simulink model "EKF_CodeOptimiert"  (Simulink 8.0)
settings: Solver=ode1  StartTime=0.0  StopTime=Inf  FixedStep=0.001  RelTol=1e-3
undefined symbols (not defined in the file or in its folder): d_p1, d_p2, g, l_1, l_2, m_1, m_2, m_3, P, Q, R, T, x0
settings Model: Creator=Bosselmann  LastModifiedBy=Bosselmann  BufferReuse=off
settings OptimizationCC: BlockReduction=off  OptimizeBlockIOStorage=off  BufferReuse=off  ExpressionFolding=off  LocalBlockOutputs=off
settings HardwareCC: ProdIntDivRoundTo=Zero  ProdEndianess=BigEndian  ProdHWDeviceType=Generic->Custom  TargetIntDivRoundTo=Zero  TargetEndianess=BigEndian  TargetHWDeviceType=Generic->Custom
settings RTWCC: SystemTargetFile=rti1401.tlc  MakeCommand=make_rti  TemplateMakefile=rti1401.tmf  Description=dSPACE DS1401 Hardware Platform  ProcessScript=rti1401_make_rtw_hook
settings STFCustomTargetCC: CodeReplacementLibrary=ANSI_C  ParMdlRefBuildCompliant=on  GeneratePreprocessorConditionals=Disable all  MatFileLogging=on  SystemTargetFile=rti1401.tlc
settings GRTTargetCC: CompOptLevelCompliant=off  ConcurrentExecutionCompliant=off  CombineOutputUpdateFcns=off  GRTInterface=on
settings CustomProperty: DataType=RTWOptions_EnumType_C__Program Files (x86)_dSPACE RCPHIL 74_MATLAB_RTI_RTI1401_TLC_rti1401_1InitialSimState  Value=RUN
settings EnumStrPairs: String=RUN

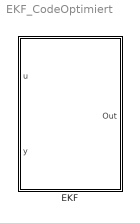
== system EKF_CodeOptimiert ==
  EKF : Subsystem

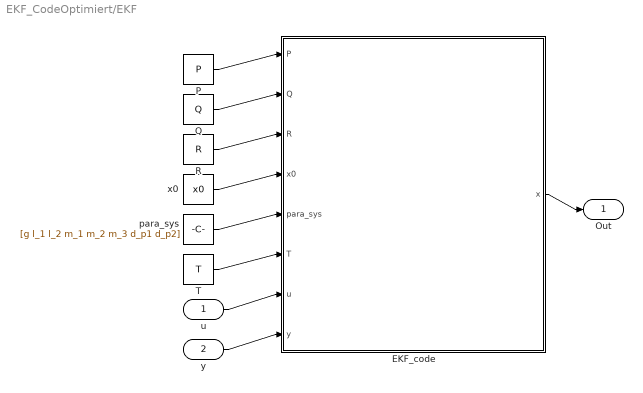
== system EKF_CodeOptimiert/EKF ==
  u : Inport
  y : Inport  Port=2
  EKF_code : MATLAB Function  TreatAsAtomicUnit=on
  P : Constant  Value=P
  Q : Constant  Value=Q
  R : Constant  Value=R
  T : Constant  Value=T
  para_sys : Constant  Value=[g l_1 l_2 m_1 m_2 m_3 d_p1 d_p2]
  x0 : Constant  Value=x0
  Out : Outport
  wires:
  P/1 -> EKF_code/1(P)
  Q/1 -> EKF_code/2(Q)
  R/1 -> EKF_code/3(R)
  x0/1 -> EKF_code/4(x0)
  para_sys/1 -> EKF_code/5(para_sys)
  T/1 -> EKF_code/6(T)
  u/1 -> EKF_code/7(u)
  y/1 -> EKF_code/8(y)
  EKF_code/1(x) -> Out/1

== matlab function EKF/EKF_code ==
  data: P input double; Q input double; R input double; x0 input double; para_sys input double; T input double; u input double; y input double; x output double
function x  = extended_kalman_filter(P, Q, R, x0, para_sys, T, u, y)
% Extended Kalman Filter (EKF) fuer nichtlineare Systeme
% Das Extended Kalman Filter praediziert den Zustand eines nichtlinearen
% Systems durch Linearisierung im Arbeistpunkt.
% R ist die Kovarianzmatrix fuer das Messrauschen.
% Q ist die Kovarianzmatrix fuer das Prozessrauschen.
% Das Verhaeltnis von Q und R gibt die Dynamik des Filters vor.

persistent x_p P_p
% Parameter

g = para_sys(1);
l_1 = para_sys(2);
l_2 = para_sys(3);
m_1 = para_sys(4);
m_2 = para_sys(5);
m_3 = para_sys(6);
d_p1 = para_sys(7);
d_p2 = para_sys(8);

if isempty(x_p)
   x_p = x0;
   P_p = P;
   x = x_p;
else
%% Discrete Kalman filter time update equations

 x_1 = x_p(1);
 x_2 = x_p(2);
 x_3 = x_p(3);
 x_4 = x_p(4);

  t3 = x_1-x_3;
  t2 = cos(t3);
  t4 = cos(x_1);
  t5 = sin(x_1);
  t6 = sin(t3);
  t7 = l_1^2;
  t8 = x_2^2;
  t9 = m_2^2;
  t10 = cos(x_3);
  t11 = sin(x_3);
  t12 = l_2^2;
  t13 = x_4^2;
  t14 = x_1*2.0;
  t15 = t14-x_3*2.0;
  t16 = t14-x_3;
  t17 = cos(t16);
  t18 = sin(t16);
  t1 = zeros(4,1);
  t1(1,1) = x_1+T*x_2;
  t1(2,1) = x_2+(T*1.0/l_1^2*(-t2*(d_p2*l_1*x_2*1.8e1-d_p2*l_1*x_4*1.8e1+g*l_1*l_2*m_2*t11*9.0+l_1*l_2*m_2*t10*u*9.0+l_2*m_2*t6*t7*t8*9.0)-d_p1*l_2*x_2*1.2e1-d_p2*l_2*x_2*1.2e1+d_p2*l_2*x_4*1.2e1+g*l_1*l_2*m_1*t5*6.0+g*l_1*l_2*m_2*t5*1.2e1+g*l_1*l_2*m_3*t5*1.2e1+l_1*l_2*m_1*t4*u*6.0+l_1*l_2*m_2*t4*u*1.2e1+l_1*l_2*m_3*t4*u*1.2e1-l_1*m_2*t6*t12*t13*6.0))/(l_2*(m_1*4.0+m_2*1.2e1+m_3*1.2e1-m_2*t2^2*9.0));
  t1(3,1) = x_3+T*x_4;
  t1(4,1) = x_4+(T*1.0/l_2^2*(t6*(l_2*t7*t8*t9*3.6e1+l_2*m_1*m_2*t7*t8*1.2e1+l_2*m_2*m_3*t7*t8*3.6e1)+d_p2*l_1*m_1*x_2*2.4e1+d_p2*l_1*m_2*x_2*7.2e1-d_p2*l_1*m_1*x_4*2.4e1+d_p2*l_1*m_3*x_2*7.2e1-d_p2*l_1*m_2*x_4*7.2e1-d_p2*l_1*m_3*x_4*7.2e1+l_1*t9*t12*t13*sin(t15)*9.0+g*l_1*l_2*t9*t11*1.8e1-g*l_1*l_2*t9*t18*1.8e1+d_p1*l_2*m_2*t2*x_2*3.6e1+d_p2*l_2*m_2*t2*x_2*3.6e1-d_p2*l_2*m_2*t2*x_4*3.6e1+l_1*l_2*t9*t10*u*1.8e1-l_1*l_2*t9*t17*u*1.8e1+g*l_1*l_2*m_1*m_2*t11*3.0+g*l_1*l_2*m_2*m_3*t11*1.8e1-g*l_1*l_2*m_1*m_2*t18*9.0-g*l_1*l_2*m_2*m_3*t18*1.8e1+l_1*l_2*m_1*m_2*t10*u*3.0+l_1*l_2*m_2*m_3*t10*u*1.8e1-l_1*l_2*m_1*m_2*t17*u*9.0-l_1*l_2*m_2*m_3*t17*u*1.8e1))/(l_1*m_2*(m_1*8.0+m_2*1.5e1+m_3*2.4e1-m_2*cos(t15)*9.0));

x = t1;
       
        % Jacobian Matrix
  t3 = x_1-x_3;
  t2 = cos(t3);
  t4 = sin(t3);
  t5 = sin(x_1);
  t6 = l_1^2;
  t7 = x_2^2;
  t8 = t2^2;
  t9 = cos(x_1);
  t10 = 1.0/l_1^2;
  t11 = 1.0/l_2;
  t12 = m_1*4.0;
  t13 = m_2*1.2e1;
  t14 = m_3*1.2e1;
  t25 = m_2*t8*9.0;
  t15 = t12+t13+t14-t25;
  t16 = d_p2*l_1*x_2*1.8e1;
  t17 = cos(x_3);
  t18 = l_1*l_2*m_2*t17*u*9.0;
  t19 = sin(x_3);
  t20 = g*l_1*l_2*m_2*t19*9.0;
  t21 = l_2*m_2*t4*t6*t7*9.0;
  t27 = d_p2*l_1*x_4*1.8e1;
  t22 = t16+t18+t20+t21-t27;
  t23 = l_2^2;
  t24 = x_4^2;
  t26 = 1.0/t15;
  t28 = l_1*m_2*t2*t23*t24*6.0;
  t29 = 1.0/t15^2;
  t30 = d_p2*l_2*x_4*1.2e1;
  t31 = l_1*l_2*m_1*t9*u*6.0;
  t32 = l_1*l_2*m_2*t9*u*1.2e1;
  t33 = l_1*l_2*m_3*t9*u*1.2e1;
  t34 = g*l_1*l_2*m_1*t5*6.0;
  t35 = g*l_1*l_2*m_2*t5*1.2e1;
  t36 = g*l_1*l_2*m_3*t5*1.2e1;
  t37 = t30+t31+t32+t33+t34+t35+t36-t2*t22-d_p1*l_2*x_2*1.2e1-d_p2*l_2*x_2*1.2e1-l_1*m_2*t4*t23*t24*6.0;
  t38 = d_p2*l_2*1.2e1;
  t39 = x_1*2.0;
  t42 = x_3*2.0;
  t40 = t39-t42;
  t41 = m_2^2;
  t43 = sin(t40);
  t44 = t39-x_3;
  t45 = cos(t44);
  t46 = sin(t44);
  t47 = 1.0/l_1;
  t48 = 1.0/l_2^2;
  t49 = m_1*8.0;
  t50 = m_2*1.5e1;
  t51 = m_3*2.4e1;
  t52 = cos(t40);
  t59 = m_2*t52*9.0;
  t53 = t49+t50+t51-t59;
  t54 = l_2*t6*t7*t41*3.6e1;
  t55 = l_2*m_1*m_2*t6*t7*1.2e1;
  t56 = l_2*m_2*m_3*t6*t7*3.6e1;
  t57 = t54+t55+t56;
  t58 = 1.0/m_2;
  t60 = 1.0/t53;
  t61 = 1.0/t53^2;
  t62 = t4*t57;
  t63 = d_p2*l_1*m_1*x_2*2.4e1;
  t64 = d_p2*l_1*m_2*x_2*7.2e1;
  t65 = d_p2*l_1*m_3*x_2*7.2e1;
  t66 = d_p1*l_2*m_2*t2*x_2*3.6e1;
  t67 = d_p2*l_2*m_2*t2*x_2*3.6e1;
  t68 = l_1*l_2*t17*t41*u*1.8e1;
  t69 = g*l_1*l_2*t19*t41*1.8e1;
  t70 = l_1*t23*t24*t41*t43*9.0;
  t71 = l_1*l_2*m_1*m_2*t17*u*3.0;
  t72 = l_1*l_2*m_2*m_3*t17*u*1.8e1;
  t73 = g*l_1*l_2*m_1*m_2*t19*3.0;
  t74 = g*l_1*l_2*m_2*m_3*t19*1.8e1;
  t75 = t62+t63+t64+t65+t66+t67+t68+t69+t70+t71+t72+t73+t74-d_p2*l_1*m_1*x_4*2.4e1-d_p2*l_1*m_2*x_4*7.2e1-d_p2*l_1*m_3*x_4*7.2e1-g*l_1*l_2*t41*t46*1.8e1-d_p2*l_2*m_2*t2*x_4*3.6e1-l_1*l_2*t41*t45*u*1.8e1-g*l_1*l_2*m_1*m_2*t46*9.0-g*l_1*l_2*m_2*m_3*t46*1.8e1-l_1*l_2*m_1*m_2*t45*u*9.0-l_1*l_2*m_2*m_3*t45*u*1.8e1;
  t76 = t2*t57;
  t77 = d_p2*l_2*m_2*t4*x_4*3.6e1;
  t78 = l_1*t23*t24*t41*t52*1.8e1;
  t79 = d_p2*l_1*m_1*2.4e1;
  t80 = d_p2*l_1*m_2*7.2e1;
  t81 = d_p2*l_1*m_3*7.2e1;
  t82 = d_p2*l_2*m_2*t2*3.6e1;
  t1 = zeros(4,4);
  t1(1,1) = 1.0;
  t1(1,2) = T;
  t1(2,1) = -T*t10*t11*t26*(t28-t4*t22-g*l_1*l_2*m_1*t9*6.0-g*l_1*l_2*m_2*t9*1.2e1-g*l_1*l_2*m_3*t9*1.2e1+l_1*l_2*m_1*t5*u*6.0+l_1*l_2*m_2*t5*u*1.2e1+l_1*l_2*m_3*t5*u*1.2e1+l_2*m_2*t6*t7*t8*9.0)-T*m_2*t2*t4*t10*t11*t29*t37*1.8e1;
  t1(2,2) = -T*t10*t11*t26*(t38+d_p1*l_2*1.2e1+t2*(d_p2*l_1*1.8e1+l_2*m_2*t4*t6*x_2*1.8e1))+1.0;
  t1(2,3) = T*t10*t11*t26*(t28-t4*t22+t2*(g*l_1*l_2*m_2*t17*-9.0+l_1*l_2*m_2*t19*u*9.0+l_2*m_2*t2*t6*t7*9.0))+T*m_2*t2*t4*t10*t11*t29*t37*1.8e1;
  t1(2,4) = T*t10*t11*t26*(t38+d_p2*l_1*t2*1.8e1-l_1*m_2*t4*t23*x_4*1.2e1);
  t1(3,3) = 1.0;
  t1(3,4) = T;
  t1(4,1) = T*t47*t48*t58*t60*(t76+t77+t78-g*l_1*l_2*t41*t45*3.6e1-d_p1*l_2*m_2*t4*x_2*3.6e1-d_p2*l_2*m_2*t4*x_2*3.6e1+l_1*l_2*t41*t46*u*3.6e1-g*l_1*l_2*m_1*m_2*t45*1.8e1-g*l_1*l_2*m_2*m_3*t45*3.6e1+l_1*l_2*m_1*m_2*t46*u*1.8e1+l_1*l_2*m_2*m_3*t46*u*3.6e1)-T*t43*t47*t48*t61*t75*1.8e1;
  t1(4,2) = T*t47*t48*t58*t60*(t79+t80+t81+t82+t4*(l_2*t6*t41*x_2*7.2e1+l_2*m_1*m_2*t6*x_2*2.4e1+l_2*m_2*m_3*t6*x_2*7.2e1)+d_p1*l_2*m_2*t2*3.6e1);
  t1(4,3) = -T*t47*t48*t58*t60*(t76+t77+t78-g*l_1*l_2*t17*t41*1.8e1-g*l_1*l_2*t41*t45*1.8e1-d_p1*l_2*m_2*t4*x_2*3.6e1-d_p2*l_2*m_2*t4*x_2*3.6e1+l_1*l_2*t19*t41*u*1.8e1+l_1*l_2*t41*t46*u*1.8e1-g*l_1*l_2*m_1*m_2*t17*3.0-g*l_1*l_2*m_2*m_3*t17*1.8e1-g*l_1*l_2*m_1*m_2*t45*9.0-g*l_1*l_2*m_2*m_3*t45*1.8e1+l_1*l_2*m_1*m_2*t19*u*3.0+l_1*l_2*m_2*m_3*t19*u*1.8e1+l_1*l_2*m_1*m_2*t46*u*9.0+l_1*l_2*m_2*m_3*t46*u*1.8e1)+T*t43*t47*t48*t61*t75*1.8e1;
  t1(4,4) = -T*t47*t48*t58*t60*(t79+t80+t81+t82-l_1*t23*t41*t43*x_4*1.8e1)+1.0;

A = t1;
C = [1 0 0 0];

%% Discrete Kalman filter measurement update equations
P   = A * P_p * A' + Q;
K   = P * C'/( C * P * C' + R);
x   = x + (K * (y - C * x));
P_p  = (eye(size(A)) - K * C) * P;
x_p  = x;
end
